simulink model "DCT"  (R2022a)
settings: Solver=VariableStepAuto  StartTime=0.0  StopTime=0  RelTol=1e-3
undefined symbols (not defined in the file or in its folder): gray, M, N, sz
libraries: vipmisc x9, visiontransforms x6, visionconversions x1, visionsources x1, deeplib x1, visiongeotforms x1
settings Model: Creator=The MathWorks, Inc.  LastModifiedBy=wzx14
settings DebuggingCC: UnconnectedInputMsg=warning  UnconnectedOutputMsg=warning  UnconnectedLineMsg=warning
settings RTWCC: DLArmComputeVersion=19.05

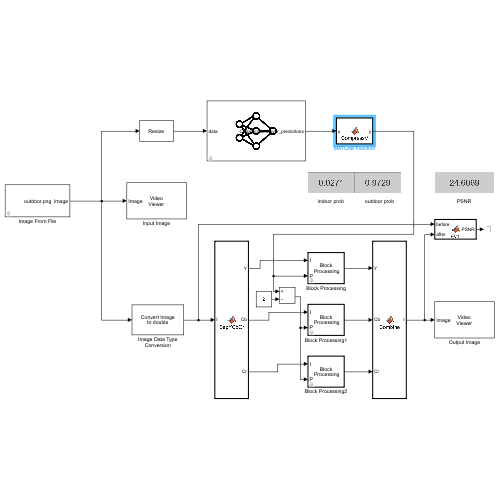
[thumbnail: Simulink's stored preview of the top-level diagram]
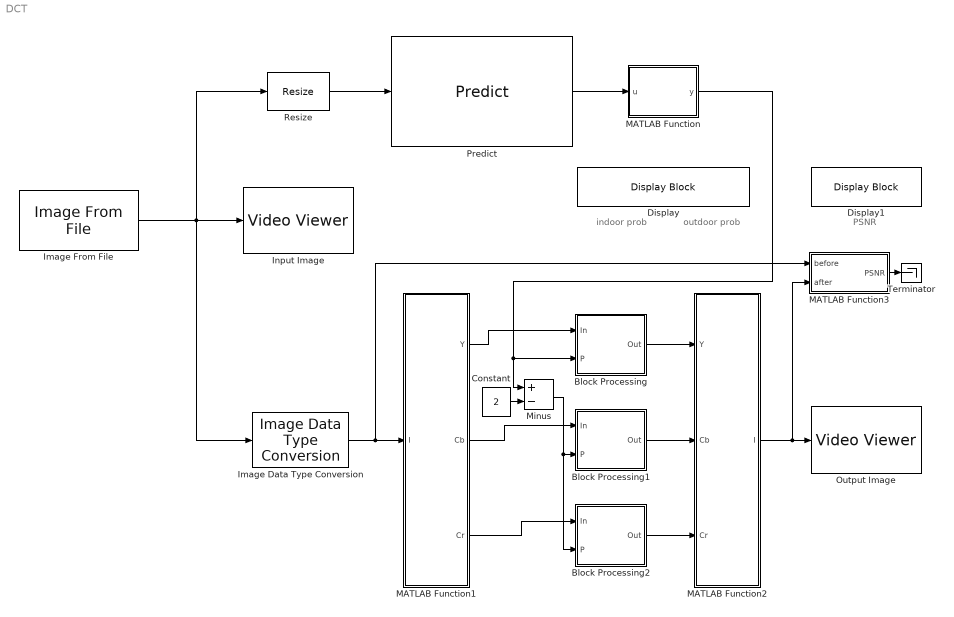
== system DCT ==
  note: outdoor prob
  note: indoor prob
  note: PSNR
  Block Processing : Subsystem  TreatAsAtomicUnit=on  mask(Block Processing){NumI=1, ParamPort=on, NumO=1, Blocksize={[8 8]}, Overlapsize={[0 0]}, Traverse=Row-wise}
      mask prompts: NumI "vision:masks:NumberOfInputs"; ParamPort "vision:masks:AddPortToSupplySubsystemParam"; NumO "vision:masks:NumberOfOutputs"; Blocksize "vision:masks:BlockSize"; Overlapsize "vision:masks:OverlapSize"; Traverse "vision:masks:TraverseOrder"
      mask help: vision:masks:BlockProcessingDescription
      mask init:
      | errmsg = vipblkblockproc(gcbh, NumI, NumO, Blocksize, Overlapsize, Traverse, ParamPort);
      | error(errmsg);
      settings: CopyFcn=set_param(gcb,'LinkStatus','none');
      mask Help: eval('helpview(fullfile(docroot,''toolbox'',''vision'',''vision.map''),''visionblockprocessing'')');
      mask TypeOptions Traverse: vision:masks:Rowwise | vision:masks:Columnwise
      mask DialogControl NumI Prompt: Number of inputs:
      mask DialogControl ParamPort Prompt: Add port to supply subsystem parameters
      mask DialogControl NumO Prompt: Number of outputs:
      mask DialogControl Blocksize Prompt: Block size:
      mask DialogControl Overlapsize Prompt: Overlap size:
      mask DialogControl Traverse Prompt: Traverse order:
      mask DialogControl subsystemGrpBox Prompt: vision:masks:Subsystem
      mask DialogControl subsystemText Prompt: vision:masks:ClickTheOpenSubsystemButton
      mask DialogControl openSubsystem Prompt: vision:masks:OpenSubsystem
      mask DialogControl openSubsystem Callback: Opensubsystem(gcbh)
      mask Display:
      | disp('Block\n Processing');
      | 
      | if ((NumI == 1) && ParamPort)
      |     port_label('input', 1, 'I');
      | end
      | 
      | if (NumI > 1)
      |     for (i = 1:NumI)
      |         port_label('input', i, ['I' int2str(i)]);
      |     end
      | end
      | 
      | if (ParamPort)
      |     port_label('input', NumI+1, 'P');
      | end
  Block Processing1 : Subsystem  TreatAsAtomicUnit=on  mask(Block Processing){NumI=1, ParamPort=on, NumO=1, Blocksize={[8 8]}, Overlapsize={[0 0]}, Traverse=Row-wise}
      mask prompts: NumI "vision:masks:NumberOfInputs"; ParamPort "vision:masks:AddPortToSupplySubsystemParam"; NumO "vision:masks:NumberOfOutputs"; Blocksize "vision:masks:BlockSize"; Overlapsize "vision:masks:OverlapSize"; Traverse "vision:masks:TraverseOrder"
      mask help: vision:masks:BlockProcessingDescription
      mask init:
      | errmsg = vipblkblockproc(gcbh, NumI, NumO, Blocksize, Overlapsize, Traverse, ParamPort);
      | error(errmsg);
      settings: CopyFcn=set_param(gcb,'LinkStatus','none');
      mask Help: eval('helpview(fullfile(docroot,''toolbox'',''vision'',''vision.map''),''visionblockprocessing'')');
      mask TypeOptions Traverse: vision:masks:Rowwise | vision:masks:Columnwise
      mask DialogControl NumI Prompt: Number of inputs:
      mask DialogControl ParamPort Prompt: Add port to supply subsystem parameters
      mask DialogControl NumO Prompt: Number of outputs:
      mask DialogControl Blocksize Prompt: Block size:
      mask DialogControl Overlapsize Prompt: Overlap size:
      mask DialogControl Traverse Prompt: Traverse order:
      mask DialogControl subsystemGrpBox Prompt: vision:masks:Subsystem
      mask DialogControl subsystemText Prompt: vision:masks:ClickTheOpenSubsystemButton
      mask DialogControl openSubsystem Prompt: vision:masks:OpenSubsystem
      mask DialogControl openSubsystem Callback: Opensubsystem(gcbh)
      mask Display:
      | disp('Block\n Processing');
      | 
      | if ((NumI == 1) && ParamPort)
      |     port_label('input', 1, 'I');
      | end
      | 
      | if (NumI > 1)
      |     for (i = 1:NumI)
      |         port_label('input', i, ['I' int2str(i)]);
      |     end
      | end
      | 
      | if (ParamPort)
      |     port_label('input', NumI+1, 'P');
      | end
  Block Processing2 : Subsystem  TreatAsAtomicUnit=on  mask(Block Processing){NumI=1, ParamPort=on, NumO=1, Blocksize={[8 8]}, Overlapsize={[0 0]}, Traverse=Row-wise}
      mask prompts: NumI "vision:masks:NumberOfInputs"; ParamPort "vision:masks:AddPortToSupplySubsystemParam"; NumO "vision:masks:NumberOfOutputs"; Blocksize "vision:masks:BlockSize"; Overlapsize "vision:masks:OverlapSize"; Traverse "vision:masks:TraverseOrder"
      mask help: vision:masks:BlockProcessingDescription
      mask init:
      | errmsg = vipblkblockproc(gcbh, NumI, NumO, Blocksize, Overlapsize, Traverse, ParamPort);
      | error(errmsg);
      settings: CopyFcn=set_param(gcb,'LinkStatus','none');
      mask Help: eval('helpview(fullfile(docroot,''toolbox'',''vision'',''vision.map''),''visionblockprocessing'')');
      mask TypeOptions Traverse: vision:masks:Rowwise | vision:masks:Columnwise
      mask DialogControl NumI Prompt: Number of inputs:
      mask DialogControl ParamPort Prompt: Add port to supply subsystem parameters
      mask DialogControl NumO Prompt: Number of outputs:
      mask DialogControl Blocksize Prompt: Block size:
      mask DialogControl Overlapsize Prompt: Overlap size:
      mask DialogControl Traverse Prompt: Traverse order:
      mask DialogControl subsystemGrpBox Prompt: vision:masks:Subsystem
      mask DialogControl subsystemText Prompt: vision:masks:ClickTheOpenSubsystemButton
      mask DialogControl openSubsystem Prompt: vision:masks:OpenSubsystem
      mask DialogControl openSubsystem Callback: Opensubsystem(gcbh)
      mask Display:
      | disp('Block\n Processing');
      | 
      | if ((NumI == 1) && ParamPort)
      |     port_label('input', 1, 'I');
      | end
      | 
      | if (NumI > 1)
      |     for (i = 1:NumI)
      |         port_label('input', i, ['I' int2str(i)]);
      |     end
      | end
      | 
      | if (ParamPort)
      |     port_label('input', NumI+1, 'P');
      | end
  Constant : Constant  Value=2
  Display : DisplayBlock  LabelPosition=Hide  Transparency=1
  Display1 : DisplayBlock  LabelPosition=Hide  Transparency=1
  Image Data Type Conversion : visionconversions/Image Data Type Conversion  outDT=double  isSigned=on  wordLen=16  numFracBits=0
      settings: SourceProductBaseCode=VP
  Image From File : visionsources/Image From File  Tag=vipblks_nd  FileName=C:\Users\wzx14\OneDrive\DSP_Lab\ResNet-50 Based Adaptive 2D-DCT Compression\Simulink_DCT\outdoor.png  Ts=inf  imagePorts=One multidimensional signal  OutPortLabels=R|G|B  ImageDataType=Inherit from input image  sdImageDataType=uint(8)  Signed=on  WordLength=16  FractionLengthMode=User-defined  FractionLength=15
  Input Image : VideoViewer  colormapValue=gray(256)  FigPos=[279.666666666667 1253.33333333333 1027.33333333333 659.333333333333]
  MATLAB Function : MATLAB Function  TreatAsAtomicUnit=on
  MATLAB Function1 : MATLAB Function  TreatAsAtomicUnit=on
  MATLAB Function2 : MATLAB Function  TreatAsAtomicUnit=on
  MATLAB Function3 : MATLAB Function  TreatAsAtomicUnit=on
  Minus : Sum  Inputs=+-
  Output Image : VideoViewer  colormapValue=gray(256)  FigPos=[1435 1347.33333333333 1120 750]
  Predict : deeplib/Predict  Network=Network from MAT-file  NetworkFunction=squeezenet  NetworkFilePath=C:\Users\wzx14\OneDrive\DSP_Lab\ResNet-50 Based Adaptive 2D-DCT Compression\Simulink_DCT\trainedNetwork_224x224.mat  MiniBatchSize=128  InputDataFormats={ '', '' }  Predictions=on  Activations={}  ForceInterpretedSim=off  EnableDLNetwork=on
      settings: SourceProductBaseCode=NN
  Resize : visiongeotforms/Resize  specify=Number of output rows and columns  rfactor=[96 96]  outCols=25  outRows=25  outRowsCols=[224 224]  interp_method=Lanczos3  antialias=on  useROI=off  roiFlag=off  roundingMode=Nearest  overflowMode=on  prodOutputMode=Binary point scaling  prodOutputWordLength=32  prodOutputFracLength=10
      settings: SourceProductBaseCode=VP
  Terminator : Terminator
  wires:
  Image From File/1 -> Image Data Type Conversion/1, Resize/1, Input Image/1
  MATLAB Function/1(y) -> Block Processing/2(P), Minus/1
  MATLAB Function2/1(I) -> MATLAB Function3/2(after), Output Image/1
  Block Processing/1(Out) -> MATLAB Function2/1(Y)
  Block Processing1/1(Out) -> MATLAB Function2/2(Cb)
  Block Processing2/1(Out) -> MATLAB Function2/3(Cr)
  Image Data Type Conversion/1 -> MATLAB Function3/1(before), MATLAB Function1/1(I)
  MATLAB Function1/1(Y) -> Block Processing/1(In)
  MATLAB Function1/2(Cb) -> Block Processing1/1(In)
  MATLAB Function1/3(Cr) -> Block Processing2/1(In)
  Constant/1 -> Minus/2
  Minus/1 -> Block Processing2/2(P), Block Processing1/2(P)
  Resize/1 -> Predict/1
  Predict/1 -> MATLAB Function/1(u)
  MATLAB Function3/1(PSNR) -> Terminator/1

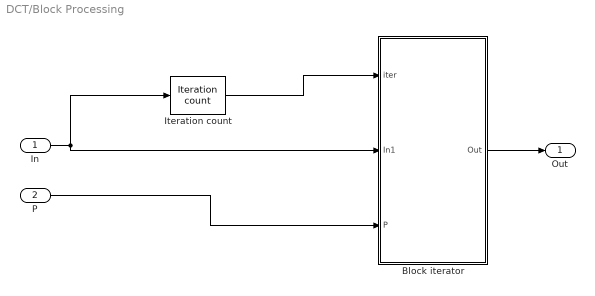
== system DCT/Block Processing ==
  In : Inport
  P : Inport  Port=2
  Block iterator : Subsystem
      settings: CopyFcn=set_param(gcb,'ReferenceBlock','');
  Iteration count : vipmisc/Iteration count  NumI=NumI  blksize={[8 8]}  ovlpsize={[0 0]}
      settings: SourceProductBaseCode=VP
  Out : Outport  VectorParamsAs1DForOutWhenUnconnected=off
  wires:
  Iteration count/1 -> Block iterator/1(iter)
  In/1 -> Iteration count/1, Block iterator/2(In1)
  Block iterator/1(Out) -> Out/1
  P/1 -> Block iterator/3(P)

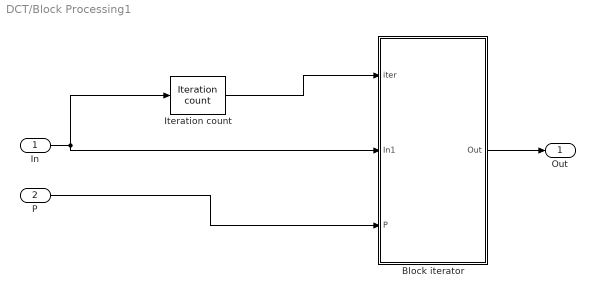
== system DCT/Block Processing1 ==
  In : Inport
  P : Inport  Port=2
  Block iterator : Subsystem
      settings: CopyFcn=set_param(gcb,'ReferenceBlock','');
  Iteration count : vipmisc/Iteration count  NumI=NumI  blksize={[8 8]}  ovlpsize={[0 0]}
      settings: SourceProductBaseCode=VP
  Out : Outport  VectorParamsAs1DForOutWhenUnconnected=off
  wires:
  Iteration count/1 -> Block iterator/1(iter)
  In/1 -> Iteration count/1, Block iterator/2(In1)
  Block iterator/1(Out) -> Out/1
  P/1 -> Block iterator/3(P)

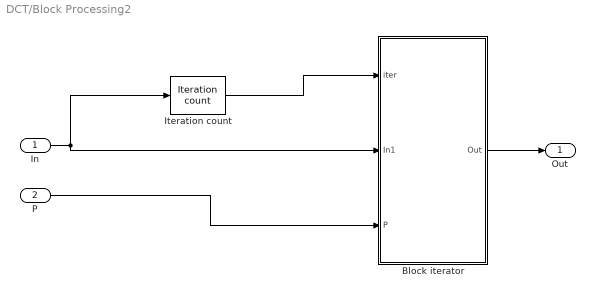
== system DCT/Block Processing2 ==
  In : Inport
  P : Inport  Port=2
  Block iterator : Subsystem
      settings: CopyFcn=set_param(gcb,'ReferenceBlock','');
  Iteration count : vipmisc/Iteration count  NumI=NumI  blksize={[8 8]}  ovlpsize={[0 0]}
      settings: SourceProductBaseCode=VP
  Out : Outport  VectorParamsAs1DForOutWhenUnconnected=off
  wires:
  Iteration count/1 -> Block iterator/1(iter)
  In/1 -> Iteration count/1, Block iterator/2(In1)
  Block iterator/1(Out) -> Out/1
  P/1 -> Block iterator/3(P)

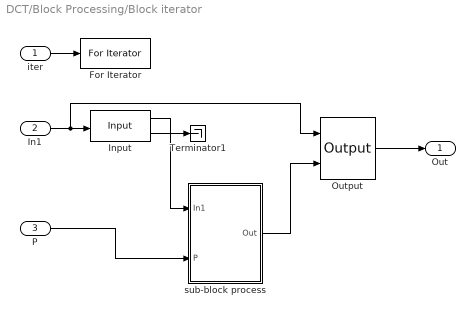
== system DCT/Block Processing/Block iterator ==
  iter : Inport
  In1 : Inport  Port=2
  P : Inport  Port=3
  For Iterator : ForIterator  IterationSource=external  IterationLimit=(sz(1)/M)*(sz(2)/N)  ShowIterationPort=off  IndexMode=Zero-based  IterationVariableDataType=double
  Input : vipmisc/Input  Blocksize=Blocksize{1}  Overlapsize=Overlapsize{1}  tverse=Row-wise
      settings: SourceProductBaseCode=VP
  Output : vipmisc/Output  Blocksize=Blocksize{1}  Overlapsize=Overlapsize{1}  tverse=Row-wise
      settings: SourceProductBaseCode=VP
  Terminator1 : Terminator
  sub-block process : Subsystem
  Out : Outport  VectorParamsAs1DForOutWhenUnconnected=off
  wires:
  Input/1 -> sub-block process/1(In1)
  iter/1 -> For Iterator/1
  In1/1 -> Input/1, Output/1
  Output/1 -> Out/1
  sub-block process/1(Out) -> Output/2
  P/1 -> sub-block process/2(P)
  Input/2 -> Terminator1/1

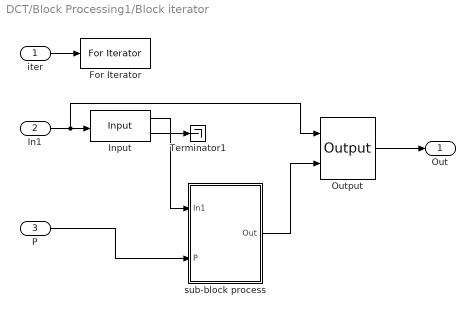
== system DCT/Block Processing1/Block iterator ==
  iter : Inport
  In1 : Inport  Port=2
  P : Inport  Port=3
  For Iterator : ForIterator  IterationSource=external  IterationLimit=(sz(1)/M)*(sz(2)/N)  ShowIterationPort=off  IndexMode=Zero-based  IterationVariableDataType=double
  Input : vipmisc/Input  Blocksize=Blocksize{1}  Overlapsize=Overlapsize{1}  tverse=Row-wise
      settings: SourceProductBaseCode=VP
  Output : vipmisc/Output  Blocksize=Blocksize{1}  Overlapsize=Overlapsize{1}  tverse=Row-wise
      settings: SourceProductBaseCode=VP
  Terminator1 : Terminator
  sub-block process : Subsystem
  Out : Outport  VectorParamsAs1DForOutWhenUnconnected=off
  wires:
  Input/1 -> sub-block process/1(In1)
  iter/1 -> For Iterator/1
  In1/1 -> Input/1, Output/1
  Output/1 -> Out/1
  sub-block process/1(Out) -> Output/2
  P/1 -> sub-block process/2(P)
  Input/2 -> Terminator1/1

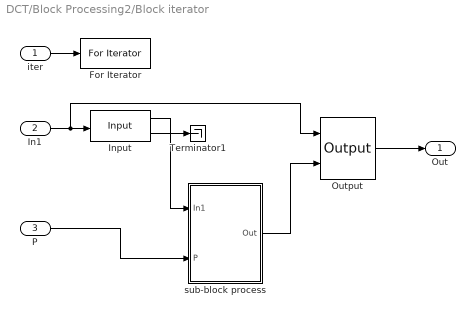
== system DCT/Block Processing2/Block iterator ==
  iter : Inport
  In1 : Inport  Port=2
  P : Inport  Port=3
  For Iterator : ForIterator  IterationSource=external  IterationLimit=(sz(1)/M)*(sz(2)/N)  ShowIterationPort=off  IndexMode=Zero-based  IterationVariableDataType=double
  Input : vipmisc/Input  Blocksize=Blocksize{1}  Overlapsize=Overlapsize{1}  tverse=Row-wise
      settings: SourceProductBaseCode=VP
  Output : vipmisc/Output  Blocksize=Blocksize{1}  Overlapsize=Overlapsize{1}  tverse=Row-wise
      settings: SourceProductBaseCode=VP
  Terminator1 : Terminator
  sub-block process : Subsystem
  Out : Outport  VectorParamsAs1DForOutWhenUnconnected=off
  wires:
  Input/1 -> sub-block process/1(In1)
  iter/1 -> For Iterator/1
  In1/1 -> Input/1, Output/1
  Output/1 -> Out/1
  sub-block process/1(Out) -> Output/2
  P/1 -> sub-block process/2(P)
  Input/2 -> Terminator1/1

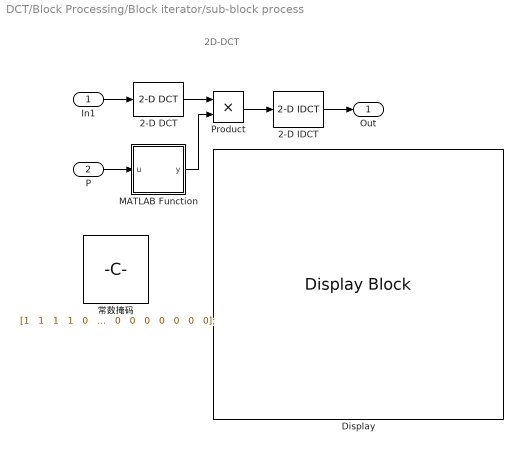
== system DCT/Block Processing/Block iterator/sub-block process ==
  note: 2D-DCT
  In1 : Inport
  P : Inport  Port=2
  2-D DCT : visiontransforms/2-D DCT  CompMethod=Table lookup  Dimension=0  TableOpt=Speed  BitRevOrder=off  SkipNorm=off  firstCoeffLastDataTypeStr=Inherit: Same word length as input  roundingMode=Floor  overflowMode=off  firstCoeffDataTypeStr=Inherit: Same word length as input  outputMin=[]  outputMax=[]
      settings: SourceProductBaseCode=VP
  2-D IDCT : visiontransforms/2-D IDCT  CompMethod=Table lookup  Dimension=0  TableOpt=Speed  BitRevOrder=off  SkipNorm=off  firstCoeffLastDataTypeStr=Inherit: Same word length as input  roundingMode=Floor  overflowMode=off  firstCoeffDataTypeStr=Inherit: Same word length as input  outputMin=[]  outputMax=[]
      settings: SourceProductBaseCode=VP
  Display : DisplayBlock  LabelPosition=Hide  Transparency=1
  MATLAB Function : MATLAB Function  TreatAsAtomicUnit=on
  Product : Product
  常数掩码 : Constant  Value=|  VectorParams1D=off
      | [1   1   1   1   0   0   0   0; 1   1   1   0   0   0   0   0
      | ; 1   1   0   0   0   0   0   0; 1   0   0   0   0   0   0   0
      | ; 0   0   0   0   0   0   0   0
      | ;  0   0   0   0   0   0   0   0
      | ; 0   0   0   0   0   0   0   0;  0   0   0   0   0   0   0   0];
  Out : Outport  VectorParamsAs1DForOutWhenUnconnected=off
  wires:
  In1/1 -> 2-D DCT/1
  2-D DCT/1 -> Product/1
  Product/1 -> 2-D IDCT/1
  2-D IDCT/1 -> Out/1
  MATLAB Function/1(y) -> Product/2
  P/1 -> MATLAB Function/1(u)

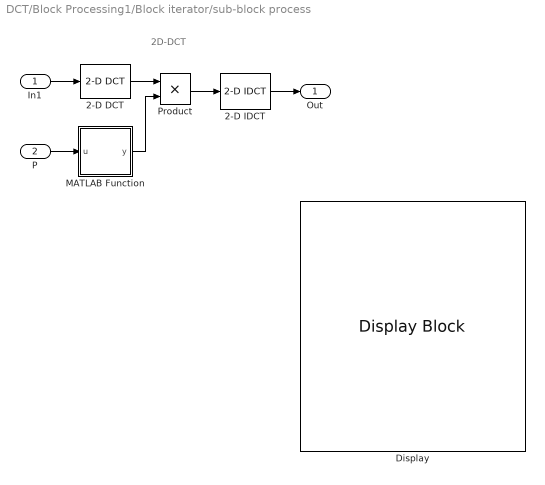
== system DCT/Block Processing1/Block iterator/sub-block process ==
  note: 2D-DCT
  In1 : Inport
  P : Inport  Port=2
  2-D DCT : visiontransforms/2-D DCT  CompMethod=Table lookup  Dimension=0  TableOpt=Speed  BitRevOrder=off  SkipNorm=off  firstCoeffLastDataTypeStr=Inherit: Same word length as input  roundingMode=Floor  overflowMode=off  firstCoeffDataTypeStr=Inherit: Same word length as input  outputMin=[]  outputMax=[]
      settings: SourceProductBaseCode=VP
  2-D IDCT : visiontransforms/2-D IDCT  CompMethod=Table lookup  Dimension=0  TableOpt=Speed  BitRevOrder=off  SkipNorm=off  firstCoeffLastDataTypeStr=Inherit: Same word length as input  roundingMode=Floor  overflowMode=off  firstCoeffDataTypeStr=Inherit: Same word length as input  outputMin=[]  outputMax=[]
      settings: SourceProductBaseCode=VP
  Display : DisplayBlock  LabelPosition=Hide  Transparency=1
  MATLAB Function : MATLAB Function  TreatAsAtomicUnit=on
  Product : Product
  Out : Outport  VectorParamsAs1DForOutWhenUnconnected=off
  wires:
  In1/1 -> 2-D DCT/1
  2-D DCT/1 -> Product/1
  Product/1 -> 2-D IDCT/1
  2-D IDCT/1 -> Out/1
  MATLAB Function/1(y) -> Product/2
  P/1 -> MATLAB Function/1(u)

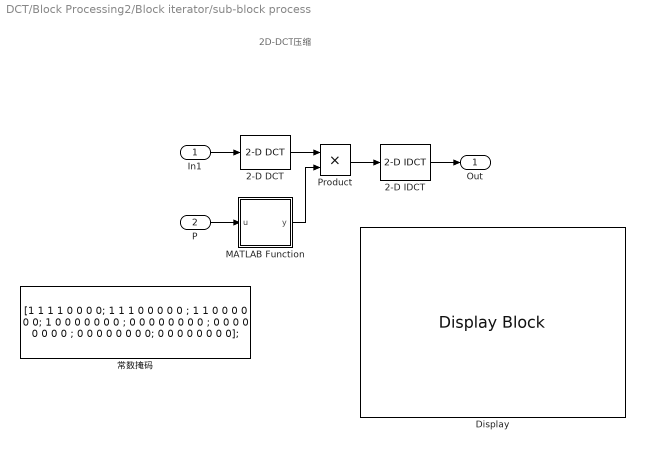
== system DCT/Block Processing2/Block iterator/sub-block process ==
  note: 2D-DCT压缩
  In1 : Inport
  P : Inport  Port=2
  2-D DCT : visiontransforms/2-D DCT  CompMethod=Table lookup  Dimension=0  TableOpt=Speed  BitRevOrder=off  SkipNorm=off  firstCoeffLastDataTypeStr=Inherit: Same word length as input  roundingMode=Floor  overflowMode=off  firstCoeffDataTypeStr=Inherit: Same word length as input  outputMin=[]  outputMax=[]
      settings: SourceProductBaseCode=VP
  2-D IDCT : visiontransforms/2-D IDCT  CompMethod=Table lookup  Dimension=0  TableOpt=Speed  BitRevOrder=off  SkipNorm=off  firstCoeffLastDataTypeStr=Inherit: Same word length as input  roundingMode=Floor  overflowMode=off  firstCoeffDataTypeStr=Inherit: Same word length as input  outputMin=[]  outputMax=[]
      settings: SourceProductBaseCode=VP
  Display : DisplayBlock  LabelPosition=Hide  Transparency=1
  MATLAB Function : MATLAB Function  TreatAsAtomicUnit=on
  Product : Product
  常数掩码 : Constant  Value=|  VectorParams1D=off
      | [1   1   1   1   0   0   0   0; 1   1   1   0   0   0   0   0
      | ; 1   1   0   0   0   0   0   0; 1   0   0   0   0   0   0   0
      | ; 0   0   0   0   0   0   0   0
      | ;  0   0   0   0   0   0   0   0
      | ; 0   0   0   0   0   0   0   0;  0   0   0   0   0   0   0   0];
  Out : Outport  VectorParamsAs1DForOutWhenUnconnected=off
  wires:
  In1/1 -> 2-D DCT/1
  2-D DCT/1 -> Product/1
  Product/1 -> 2-D IDCT/1
  2-D IDCT/1 -> Out/1
  MATLAB Function/1(y) -> Product/2
  P/1 -> MATLAB Function/1(u)

== matlab function DCT/Block Processing/Block iterator/sub-block process/MATLAB Function ==
  data: u input; y output
function y = Mask(u)

y = zeros([8,8]);
for i=1:min(u,8)
    for j=1:min(u-i+1,8)
        y(i,j)=1;
    end
end

== matlab function DCT/MATLAB Function ==
  data: u input; y output
function y = CompressV(u)

if u(1)>0.5
    y=12;
else
    y=6;
end

== matlab function DCT/MATLAB Function1 ==
  data: I input; Y output; Cb output; Cr output
function [Y,Cb,Cr] = SepYCbCr(I)

[Y,Cb,Cr]=imsplit(rgb2ycbcr(I));

== matlab function DCT/Block Processing1/Block iterator/sub-block process/MATLAB Function ==
  data: u input; y output
function y = Mask(u)

y = zeros([8,8]);
for i=1:min(u,8)
    for j=1:min(u-i+1,8)
        y(i,j)=1;
    end
end

== matlab function DCT/Block Processing2/Block iterator/sub-block process/MATLAB Function ==
  data: u input; y output
function y = Mask(u)

y = zeros([8,8]);
for i=1:min(u,8)
    for j=1:min(u-i+1,8)
        y(i,j)=1;
    end
end

== matlab function DCT/MATLAB Function2 ==
  data: Y input; I output; Cb input; Cr input
function I = Combine(Y,Cb,Cr)

I=ycbcr2rgb(cat(3, Y, Cb, Cr));

== matlab function DCT/MATLAB Function3 ==
  data: before input; PSNR output; after input
function PSNR  = Eval(before,after)

PSNR=psnr(after,before);
